simulink model "Constant_Torque_Split"  (R2020a)
settings: Solver=FixedStepDiscrete  StartTime=0.0  StopTime=inf  FixedStep=0.01  RelTol=1e-3  EnableMultiTasking=on
undefined symbols (not defined in the file): VEH
settings Model: DataDictionary=System_Data_Dictionary.sldd  Creator=koshiro  LastModifiedBy=jchu
settings SolverCC: AutoInsertRateTranBlk=on
settings DataIOCC: ReturnWorkspaceOutputs=off
settings OptimizationCC: UseDivisionForNetSlopeComputation=on
settings DebuggingCC: ArithmeticOperatorsInVariantConditions=warning
settings SFSimCC: CustomCodeUndefinedFunction=UseInterfaceOnly

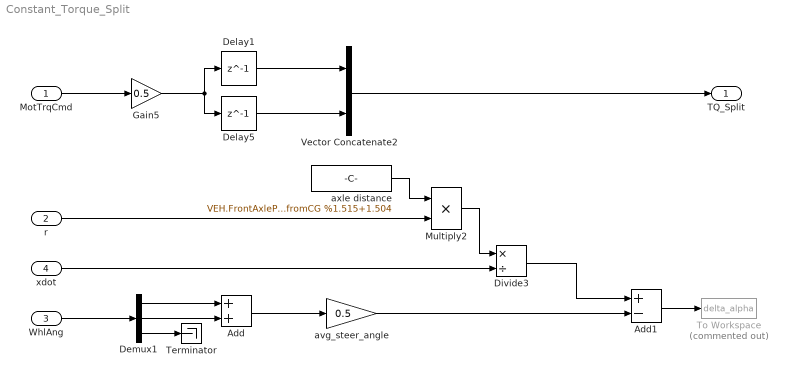
== system Constant_Torque_Split ==
  MotTrqCmd : Inport
  r : Inport  Port=2
  WhlAng : Inport  Port=3
  xdot : Inport  Port=4
  Add : Sum
  Add1 : Sum  Inputs=+-
  Delay1 : Delay  DelayLength=1  InitialCondition=0
  Delay5 : Delay  DelayLength=1  InitialCondition=0
  Demux1 : Demux  Outputs=[1 1 2]
  Divide3 : Product  Inputs=*/
  Gain5 : Gain  Gain=0.5
  Multiply2 : Product
  Terminator : Terminator
  To Workspace : ToWorkspace  Commented=on  VariableName=delta_alpha  SaveFormat=Timeseries  SampleTime=-1
  Vector Concatenate2 : Concatenate
  avg_steer_angle : Gain  Gain=0.5
  axle distance : Constant  Value=VEH.FrontAxlePositionfromCG + VEH.RearAxlePositionfromCG %1.515+1.504
  TQ_Split : Outport  VectorParamsAs1DForOutWhenUnconnected=off
  wires:
  Vector Concatenate2/1 -> TQ_Split/1
  MotTrqCmd/1 -> Gain5/1
  Delay5/1 -> Vector Concatenate2/2
  Delay1/1 -> Vector Concatenate2/1
  Gain5/1 -> Delay1/1, Delay5/1
  Demux1/2 -> Add/2
  Divide3/1 -> Add1/1
  Add/1 -> avg_steer_angle/1
  Add1/1 -> To Workspace/1
  Demux1/1 -> Add/1
  r/1 -> Multiply2/2
  axle distance/1 -> Multiply2/1
  xdot/1 -> Divide3/2
  Demux1/3 -> Terminator/1
  avg_steer_angle/1 -> Add1/2
  Multiply2/1 -> Divide3/1
  WhlAng/1 -> Demux1/1
